simulink model "lab8schema"  (R2023b)
settings: Solver=VariableStepAuto  StartTime=0.0  StopTime=30  RelTol=1e-3
undefined symbols (not defined in the file): C1, C2, K1, K2, p, P1, P2, T
libraries: checkpacklib x3, simulink x2, hdlsllib x1
settings Model: Creator=user  LastModifiedBy=user

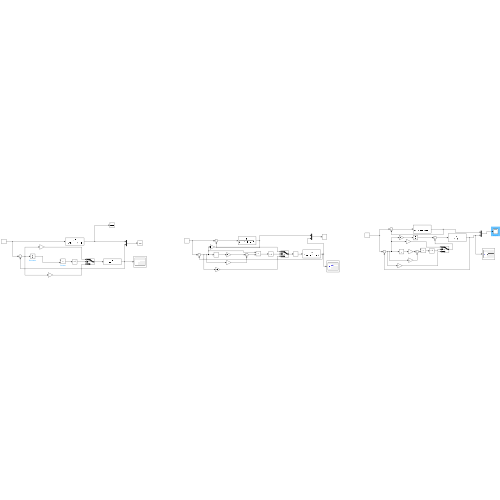
[thumbnail: Simulink's stored preview of the top-level diagram]
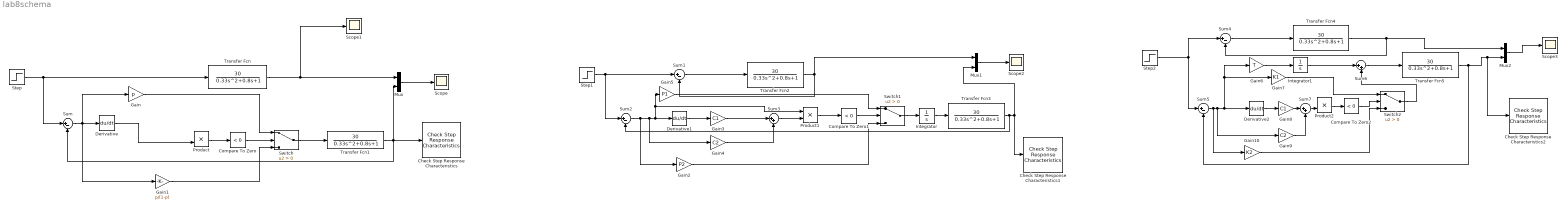
== system lab8schema ==
  Check Step Response Characteristics : checkpacklib/Check Step Response  Characteristics  InstantiateOnLoad=on  enabled=on  stopWhenAssertionFail=off  export=off  ViewDlgPos=[]  OpenViewOnLoad=off  LaunchViewOnOpen=off  TimeUnits=seconds  EnableStepResponseBound=on  InitialValue=0  FinalValue=1  StepTime=0  RiseTime=5  PercentRise=80  SettlingTime=7  PercentSettling=1  PercentOvershoot=10  PercentUndershoot=1
      settings: LibrarySourceBlock=|
      | sdolib/Model Verification/Check Step Response
      | Characteristics
  Check Step Response Characteristics1 : checkpacklib/Check Step Response  Characteristics  InstantiateOnLoad=on  enabled=on  stopWhenAssertionFail=off  export=off  ViewDlgPos=[]  OpenViewOnLoad=off  LaunchViewOnOpen=off  TimeUnits=seconds  EnableStepResponseBound=on  InitialValue=0  FinalValue=1  StepTime=0  RiseTime=5  PercentRise=80  SettlingTime=7  PercentSettling=1  PercentOvershoot=10  PercentUndershoot=1
      settings: LibrarySourceBlock=|
      | sdolib/Model Verification/Check Step Response
      | Characteristics
  Check Step Response Characteristics2 : checkpacklib/Check Step Response  Characteristics  InstantiateOnLoad=on  enabled=on  stopWhenAssertionFail=off  export=off  ViewDlgPos=[]  OpenViewOnLoad=off  LaunchViewOnOpen=off  TimeUnits=seconds  EnableStepResponseBound=on  InitialValue=0  FinalValue=1  StepTime=0  RiseTime=5  PercentRise=80  SettlingTime=7  PercentSettling=1  PercentOvershoot=10  PercentUndershoot=1
      settings: LibrarySourceBlock=|
      | sdolib/Model Verification/Check Step Response
      | Characteristics
  Compare To Zero : hdlsllib/Logic and Bit Operations/Compare To Zero  relop=<  OutDataTypeStr=boolean
  Compare To Zero1 : simulink/Logic and Bit Operations/Compare To Zero  relop=<  OutDataTypeStr=boolean
  Compare To Zero2 : simulink/Logic and Bit Operations/Compare To Zero  relop=<  OutDataTypeStr=boolean
  Derivative : Derivative
  Derivative1 : Derivative
  Derivative2 : Derivative
  Gain : Gain  Gain=p
  Gain1 : Gain  Gain=p/(1-p)
  Gain10 : Gain  Gain=K2
  Gain2 : Gain  Gain=P2
  Gain3 : Gain  Gain=C1
  Gain4 : Gain  Gain=C2
  Gain5 : Gain  Gain=P1
  Gain6 : Gain  Gain=T
  Gain7 : Gain  Gain=K1
  Gain8 : Gain  Gain=C1
  Gain9 : Gain  Gain=C2
  Integrator : Integrator
  Integrator1 : Integrator
  Mux : Mux  Inputs=2
  Mux1 : Mux  Inputs=2
  Mux2 : Mux  Inputs=2
  Product : Product
  Product1 : Product
  Product2 : Product
  Scope{,1..3} (4 alike) : Scope
  Step : Step  Time=0  SampleTime=0
  Step1 : Step  Time=0  SampleTime=0
  Step2 : Step  Time=0  SampleTime=0
  Sum{,1..2,4..5} (5 alike) : Sum  Inputs=|+-
  Sum3 : Sum  Inputs=|++
  Sum6 : Sum  Inputs=|++
  Sum7 : Sum  Inputs=|++
  Switch : Switch  Criteria=u2 > Threshold  SaturateOnIntegerOverflow=off  InputSameDT=off
  Switch1 : Switch  Criteria=u2 > Threshold  SaturateOnIntegerOverflow=off  InputSameDT=off
  Switch2 : Switch  Criteria=u2 > Threshold  SaturateOnIntegerOverflow=off  InputSameDT=off
  Transfer Fcn{,1..5} (6 alike) : TransferFcn  Numerator=[30]  Denominator=[0.33 0.8 1]
  wires:
  Step/1 -> Sum/1, Transfer Fcn/1
  Transfer Fcn/1 -> Mux/1, Scope1/1
  Mux/1 -> Scope/1
  Sum/1 -> Gain1/1, Gain/1, Derivative/1
  Derivative/1 -> Product/2
  Product/1 -> Compare To Zero/1
  Gain/1 -> Switch/1
  Compare To Zero/1 -> Switch/2
  Gain1/1 -> Switch/3
  Switch/1 -> Transfer Fcn1/1
  Transfer Fcn1/1 -> Sum/2, Mux/2, Check Step Response Characteristics/1
  Step1/1 -> Sum2/1, Sum1/1
  Sum1/1 -> Transfer Fcn2/1
  Transfer Fcn2/1 -> Mux1/1, Sum1/2
  Sum2/1 -> Gain2/1, Gain4/1, Product1/1, Gain5/1, Derivative1/1
  Derivative1/1 -> Gain3/1
  Gain3/1 -> Sum3/1
  Gain4/1 -> Sum3/2
  Sum3/1 -> Product1/2
  Product1/1 -> Compare To Zero1/1
  Gain5/1 -> Switch1/1
  Compare To Zero1/1 -> Switch1/2
  Gain2/1 -> Switch1/3
  Mux1/1 -> Scope2/1
  Transfer Fcn3/1 -> Sum2/2, Mux1/2, Check Step Response Characteristics1/1
  Switch1/1 -> Integrator/1
  Integrator/1 -> Transfer Fcn3/1
  Step2/1 -> Sum5/1, Sum4/1
  Sum4/1 -> Transfer Fcn4/1
  Transfer Fcn4/1 -> Sum4/2, Mux2/1
  Mux2/1 -> Scope3/1
  Sum5/1 -> Gain10/1, Gain9/1, Gain7/1, Gain6/1, Derivative2/1
  Gain6/1 -> Integrator1/1
  Integrator1/1 -> Sum6/1
  Sum6/1 -> Transfer Fcn5/1
  Transfer Fcn5/1 -> Sum5/2, Check Step Response Characteristics2/1, Mux2/2
  Gain7/1 -> Switch2/1
  Switch2/1 -> Sum6/2
  Compare To Zero2/1 -> Switch2/2
  Product2/1 -> Compare To Zero2/1
  Derivative2/1 -> Gain8/1
  Gain8/1 -> Sum7/1
  Sum7/1 -> Product2/2
  Gain9/1 -> Sum7/2
  Gain10/1 -> Switch2/3
